simulink model "tek_fazli_uc_seviyeli_spwm"  (R2019b)
settings: Solver=VariableStepDiscrete  StartTime=0.0  StopTime=0.5  MaxStep=10e-5  RelTol=1e-3
libraries: powerlib x11, simulink x2, powerlib_meascontrol x1
settings Model: Creator=Monster  LastModifiedBy=Monster

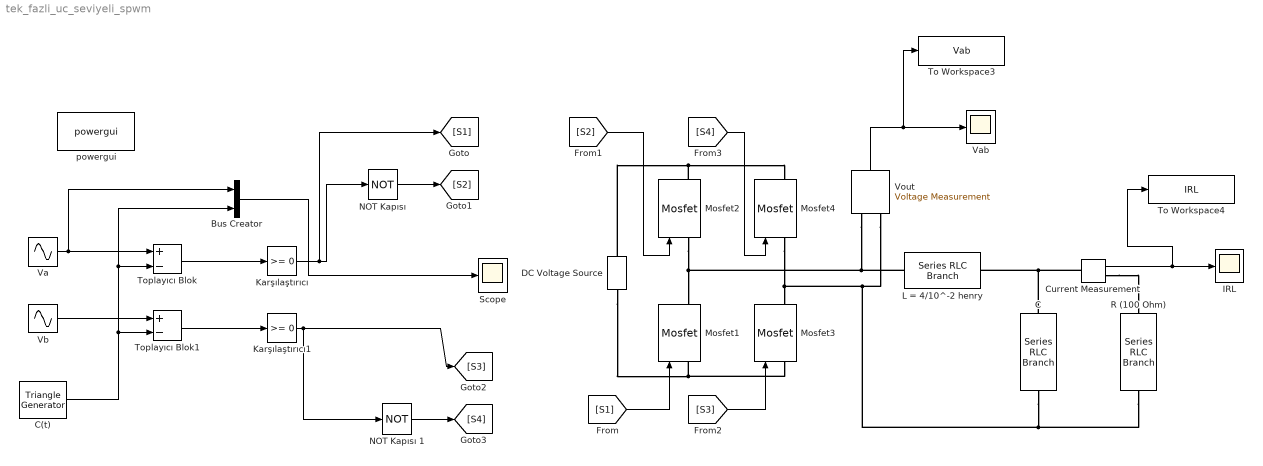
== system tek_fazli_uc_seviyeli_spwm ==
  Bus Creator : BusCreator  Inputs=2
  C : powerlib/Elements/Series RLC Branch  LConnTagsString=__new0  RConnTagsString=__new0  BranchType=C  Resistance=1  Inductance=1e-3  SetiL0=off  InitialCurrent=0  Capacitance=2.0e-5  Setx0=off  InitialVoltage=0  Measurements=None
      settings: SourceProductName=Simscape Electrical
  C(t) : powerlib_meascontrol/Pulse & Signal Generators/Triangle Generator  Freq=2000  Phase=90  Ts=0
      settings: SourceProductName=Simscape Electrical
  Current Measurement : powerlib/Measurements/Current Measurement  PhasorSimulation=off  OutputType=Complex  PSBequivalent=0
      settings: SourceProductName=Simscape Electrical
  DC Voltage Source : powerlib/Electrical Sources/DC Voltage Source  Amplitude=100  Measurements=None
      settings: SourceProductName=Simscape Electrical
  IRL : Scope
  Karşılaştırıcı : simulink/Logic and Bit Operations/Compare To Zero  relop=>=  OutDataTypeStr=boolean
  Karşılaştırıcı1 : simulink/Logic and Bit Operations/Compare To Zero  relop=>=  OutDataTypeStr=boolean
  L = 4/10^-2 henry : powerlib/Elements/Series RLC Branch  LConnTagsString=__new0  RConnTagsString=__new0  BranchType=L  Resistance=1  Inductance=4e-2  SetiL0=off  InitialCurrent=0  Capacitance=1e-6  Setx0=off  InitialVoltage=0  Measurements=None
      settings: SourceProductName=Simscape Electrical
  "Mosfet1 " : powerlib/Power Electronics/Mosfet  Ron=0.1  Lon=0  Rd=0.01  Vfd=0  IC=0  Rs=1e5  Cs=inf  Measurements=on
      settings: SourceProductName=Simscape Electrical
  "Mosfet2 " : powerlib/Power Electronics/Mosfet  Ron=0.1  Lon=0  Rd=0.01  Vfd=0  IC=0  Rs=1e5  Cs=inf  Measurements=on
      settings: SourceProductName=Simscape Electrical
  "Mosfet3 " : powerlib/Power Electronics/Mosfet  Ron=0.1  Lon=0  Rd=0.01  Vfd=0  IC=0  Rs=1e5  Cs=inf  Measurements=on
      settings: SourceProductName=Simscape Electrical
  "Mosfet4 " : powerlib/Power Electronics/Mosfet  Ron=0.1  Lon=0  Rd=0.01  Vfd=0  IC=0  Rs=1e5  Cs=inf  Measurements=on
      settings: SourceProductName=Simscape Electrical
  NOT Kapısı : Logic  Operator=NOT  IconShape=distinctive  AllPortsSameDT=off  OutDataTypeStr=boolean
  NOT Kapısı 1 : Logic  Operator=NOT  IconShape=distinctive  AllPortsSameDT=off  OutDataTypeStr=boolean
  R (100 Ohm) : powerlib/Elements/Series RLC Branch  LConnTagsString=__new0  RConnTagsString=__new0  BranchType=RL  Resistance=100  Inductance=1e-3  SetiL0=off  InitialCurrent=0  Capacitance=1e-6  Setx0=off  InitialVoltage=0  Measurements=None
      settings: SourceProductName=Simscape Electrical
  "Scope " : Scope
  To Workspace3 : ToWorkspace  VariableName=Vab  SaveFormat=Timeseries  SampleTime=-1
  To Workspace4 : ToWorkspace  VariableName=IRL  SaveFormat=Timeseries  SampleTime=-1
  Toplayıcı Blok : Sum  Inputs=+-
  Toplayıcı Blok1 : Sum  Inputs=+-
  Va : Sin  Frequency=2*pi*50  SampleTime=0
  Vab : Scope
  Vb : Sin  Frequency=2*pi*50  Phase=pi  SampleTime=0
  Vout : powerlib/Measurements/Voltage Measurement  PhasorSimulation=off  OutputType=Complex  PSBequivalent=0
      settings: SourceProductName=Simscape Electrical
  powergui : powerlib/powergui  Priority=1  SimulationMode=Discrete  SampleTime=1e-6  frequency=60  Iterations=50  frequencyindice=0  Pbase=100e6  ErrMax=1e-4  UnitsV=kV  UnitsW=MW  buscounter=0  FunctionMessages=off  echomessages=off  EnableUseOfTLC=off  CurrentSourceSwitches=off  DisableSnubberDevices=off  DisableRonSwitches=off  DisableVfSwitches=off  DisplayEquations=off  AutomaticDiscreteSolvers=off  SolverType=Tustin/Backward Euler (TBE)  Interpol=off  ExternalGateDelay=off  methode=off  Ts=100  x0status=blocks  SPID=on  SwTol=0  HookPort=off  NonlinearTolerance=1e-4  nMaxIteration=100  ContinueOnMaxIteration=off  RestoreLinks=warning  ResistiveCurrentMeasurement=off  Frange=[0:2:500]  Ylog=off  Xlog=on  ShowGrid=off  save=off  variable=ZData  structure=0  ZoomFFT=off  StartTime=0.0  cycles=1  DisplayStyle=1  fundamental=60  FreqAxis=off  MaxFrequency=1000  frequencyindicesteady=1  RmsSteady=1  display=off
      settings: SourceProductName=Simscape Electrical
  wires:
  Va/1 -> Toplayıcı Blok/1, Bus Creator/1
  Vb/1 -> Toplayıcı Blok1/1
  C(t)/1 -> Toplayıcı Blok1/2, Bus Creator/2, Toplayıcı Blok/2
  Toplayıcı Blok/1 -> Karşılaştırıcı/1
  Toplayıcı Blok1/1 -> Karşılaştırıcı1/1
  Karşılaştırıcı/1 -> [S1], NOT Kapısı/1
  Karşılaştırıcı1/1 -> NOT Kapısı 1/1, [S3]
  NOT Kapısı/1 -> [S2]
  NOT Kapısı 1/1 -> [S4]
  Vout/1 -> Vab/1, To Workspace3/1
  Current Measurement/1 -> To Workspace4/1, IRL/1
  [S2] -> "Mosfet2 "/1
  [S1] -> "Mosfet1 "/1
  [S4] -> "Mosfet4 "/1
  [S3] -> "Mosfet3 "/1
  Bus Creator/1 -> "Scope "/1
  connections:
  "Mosfet2 "/RConn1 -- DC Voltage Source/LConn1 -- "Mosfet4 "/RConn1
  "Mosfet3 "/LConn1 -- DC Voltage Source/RConn1 -- "Mosfet1 "/LConn1
  "Mosfet2 "/LConn1 -- L = 4/10^-2 henry/LConn1 -- Vout/LConn1 -- "Mosfet1 "/RConn1
  "Mosfet4 "/LConn1 -- Vout/LConn2 -- R (100 Ohm)/RConn1 -- C/RConn1 -- "Mosfet3 "/RConn1
  C/LConn1 -- L = 4/10^-2 henry/RConn1 -- Current Measurement/LConn1
  Current Measurement/RConn1 -- R (100 Ohm)/LConn1
